simulink model "IFSSIM_Chassis"  (R2025b)
settings: Solver=FixedStepDiscrete  StartTime=0  StopTime=inf  FixedStep=1/960  RelTol=1e-3
undefined symbols (not defined in the file or in its folder): IFSSIM_CoGH, IFSSIM_Ixx, IFSSIM_Iyy, IFSSIM_Izz, IFSSIM_Mass, IFSSIM_Ts
settings Model: Creator=raulmoran  LastModifiedBy=raulmoran

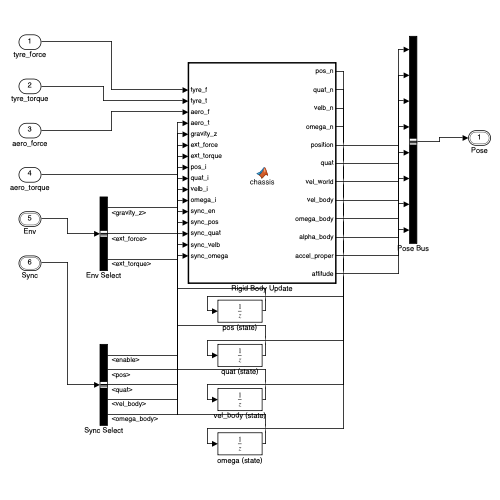
[thumbnail: Simulink's stored preview of the top-level diagram]
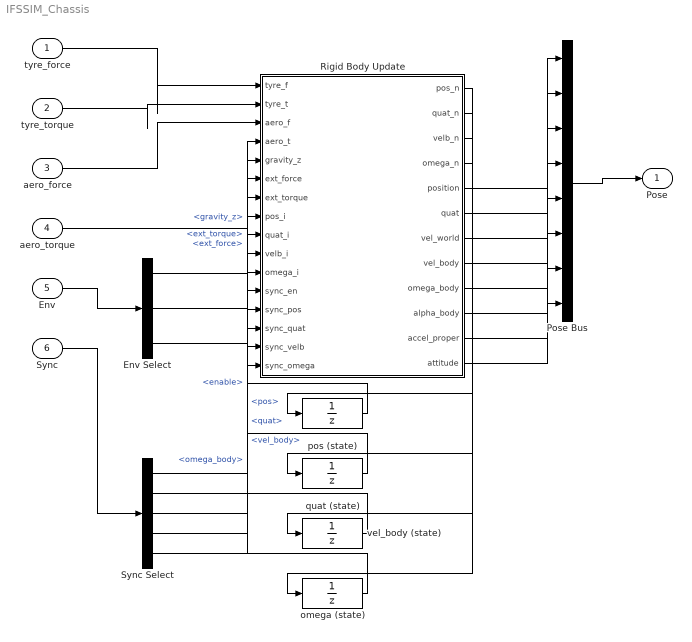
== system IFSSIM_Chassis ==
  tyre_force : Inport  PortDimensions=3
  tyre_torque : Inport  Port=2  PortDimensions=3
  aero_force : Inport  Port=3  PortDimensions=3
  aero_torque : Inport  Port=4  PortDimensions=3
  Env : Inport  Port=5  OutDataTypeStr=Bus: IFSSIM_EnvBus  BusOutputAsStruct=on
  Sync : Inport  Port=6  OutDataTypeStr=Bus: IFSSIM_SyncBus  BusOutputAsStruct=on
  Env Select : BusSelector  OutputSignals=gravity_z,ext_force,ext_torque
  Pose Bus : BusCreator  Inputs=8  OutDataTypeStr=Bus: IFSSIM_PoseBus  NonVirtualBus=on
  Rigid Body Update : MATLAB Function  TreatAsAtomicUnit=on
  Sync Select : BusSelector  OutputSignals=enable,pos,quat,vel_body,omega_body
  omega (state) : UnitDelay  InitialCondition=[0;0;0]  SampleTime=-1  HasFrameUpgradeWarning=on
  pos (state) : UnitDelay  InitialCondition=[0;0;IFSSIM_CoGH]  SampleTime=-1  HasFrameUpgradeWarning=on
  quat (state) : UnitDelay  InitialCondition=[1;0;0;0]  SampleTime=-1  HasFrameUpgradeWarning=on
  vel_body (state) : UnitDelay  InitialCondition=[0;0;0]  SampleTime=-1  HasFrameUpgradeWarning=on
  Pose : Outport  OutDataTypeStr=Bus: IFSSIM_PoseBus
  wires:
  Env/1 -> Env Select/1
  Sync/1 -> Sync Select/1
  Pose Bus/1 -> Pose/1
  tyre_force/1 -> Rigid Body Update/1(tyre_f)
  tyre_torque/1 -> Rigid Body Update/2(tyre_t)
  aero_force/1 -> Rigid Body Update/3(aero_f)
  aero_torque/1 -> Rigid Body Update/4(aero_t)
  Env Select/1 -> Rigid Body Update/5(gravity_z)  "<gravity_z>"
  Env Select/2 -> Rigid Body Update/6(ext_force)  "<ext_force>"
  Env Select/3 -> Rigid Body Update/7(ext_torque)  "<ext_torque>"
  pos (state)/1 -> Rigid Body Update/8(pos_i)
  quat (state)/1 -> Rigid Body Update/9(quat_i)
  vel_body (state)/1 -> Rigid Body Update/10(velb_i)
  omega (state)/1 -> Rigid Body Update/11(omega_i)
  Sync Select/1 -> Rigid Body Update/12(sync_en)  "<enable>"
  Sync Select/2 -> Rigid Body Update/13(sync_pos)  "<pos>"
  Sync Select/3 -> Rigid Body Update/14(sync_quat)  "<quat>"
  Sync Select/4 -> Rigid Body Update/15(sync_velb)  "<vel_body>"
  Sync Select/5 -> Rigid Body Update/16(sync_omega)  "<omega_body>"
  Rigid Body Update/1(pos_n) -> pos (state)/1
  Rigid Body Update/2(quat_n) -> quat (state)/1
  Rigid Body Update/3(velb_n) -> vel_body (state)/1
  Rigid Body Update/4(omega_n) -> omega (state)/1
  Rigid Body Update/5(position) -> Pose Bus/1
  Rigid Body Update/6(quat) -> Pose Bus/2
  Rigid Body Update/7(vel_world) -> Pose Bus/3
  Rigid Body Update/8(vel_body) -> Pose Bus/4
  Rigid Body Update/9(omega_body) -> Pose Bus/5
  Rigid Body Update/10(alpha_body) -> Pose Bus/6
  Rigid Body Update/11(accel_proper) -> Pose Bus/7
  Rigid Body Update/12(attitude) -> Pose Bus/8

== matlab function IFSSIM_Chassis/Rigid Body Update ==
  data: tyre_f input size=3; pos_n output size=3; tyre_t input size=3; aero_f input size=3; aero_t input size=3; gravity_z input size=1; ext_force input size=3; ext_torque input size=3; pos_i input size=3; quat_i input size=4; velb_i input size=3; omega_i input size=3; sync_en input size=1; sync_pos input size=3; sync_quat input size=4; sync_velb input size=3; sync_omega input size=3; quat_n output size=4; velb_n output size=3; omega_n output size=3; position output size=3; quat output size=4; vel_world output size=3; vel_body output size=3; omega_body output size=3; alpha_body output size=3; accel_proper output size=3; attitude output size=3; IFSSIM_Ts parameter size=1; IFSSIM_Mass parameter size=1; IFSSIM_Ixx parameter size=1; IFSSIM_Iyy parameter size=1; IFSSIM_Izz parameter size=1; IFSSIM_CoGH parameter size=1
function [pos_n, quat_n, velb_n, omega_n, position, quat, vel_world, vel_body, omega_body, alpha_body, accel_proper, attitude] = ...
         chassis(tyre_f, tyre_t, aero_f, aero_t, gravity_z, ext_force, ext_torque, pos_i, quat_i, velb_i, omega_i, ...
                 sync_en, sync_pos, sync_quat, sync_velb, sync_omega, IFSSIM_Ts, IFSSIM_Mass, IFSSIM_Ixx, IFSSIM_Iyy, IFSSIM_Izz, IFSSIM_CoGH)
%#codegen
% 6-DOF rigid body, Newton-Euler in the body frame, forward Euler at Ts.
%
% Frames: body is ISO 8855 / REP-103 — x forward, y LEFT, z up. World is ENU.
% Wheel order elsewhere is FL, FR, RL, RR.
%
% tyre_f / aero_f arrive in the BODY frame (they are generated by body-attached
% things). ext_force is WORLD — it comes from the platform's collision solver,
% which has no opinion about the car's orientation.
%
% The Env bus is split by a Bus Selector OUTSIDE this block rather than passed
% in whole. Two reasons: a MATLAB Function block has to infer a struct type
% through the port, which is fragile; and the selector makes the diagram show
% exactly which Env fields the chassis consumes.

% Flat workspace scalars, not IFSSIM_P.Assumed.Izz: a MATLAB Function block
% resolves workspace variables as parameters and that lookup does not reach
% into nested structs. See ifssim_load_workspace.m — still one source, still
% settings.json.
Ts = IFSSIM_Ts;
m  = IFSSIM_Mass;
I  = [IFSSIM_Ixx; IFSSIM_Iyy; IFSSIM_Izz];   % principal, diagonal

% --- state injection -------------------------------------------------
% Applied to the INCOMING state, before any dynamics. Overriding the outgoing
% state instead would look equivalent and is not: this step would still
% compute its forces and its reported acceleration from the OLD pose, so the
% caller would read a response to a state the plant is no longer in. For a
% one-step comparison against a reference that is precisely the wrong answer,
% and it is wrong by one step, which is the hardest kind of wrong to see.
%
% Normal running leaves enable at zero and nothing here executes.
if sync_en > 0.5
    pos_i   = sync_pos;
    quat_i  = sync_quat / max(norm(sync_quat), eps);
    velb_i  = sync_velb;
    omega_i = sync_omega;
end

% --- orientation ---------------------------------------------------
q = quat_i / max(norm(quat_i), eps);        % renormalise every step: forward Euler
                                        % on a quaternion drifts off the unit
                                        % sphere, and the drift is silent.
R = quat2rotm_local(q);                 % body -> world

% --- forces ----------------------------------------------------------
% Everything to the body frame first, then one sum. Mixing frames in a
% force accumulator is the classic way to get a plausible-but-wrong plant.
F_body = tyre_f + aero_f + R' * ext_force;
M_body = tyre_t + aero_t + R' * ext_torque;

% PROPER acceleration excludes gravity — it is what an accelerometer reads.
% Publishing this directly is the point: the simulator currently finite-
% differences a world velocity and bolts +g on, which is where the missing
% Coriolis terms in the EKF came from.
accel_proper = F_body / m;

% Gravity acts on the body but is NOT felt by an accelerometer, so it enters
% the equation of motion after accel_o has been taken.
g_body = R' * [0; 0; gravity_z];

% --- rigid body ------------------------------------------------------
% v_dot = F/m + g - omega x v      (Coriolis term: body-frame rates are not
%                                   inertial, and dropping this is exactly the
%                                   bug that made vy drift during cornering)
vdot  = accel_proper + g_body - cross(omega_i, velb_i);

% I*omega_dot = M - omega x (I*omega)   (gyroscopic coupling)
Iw    = I .* omega_i;
alpha_body = (M_body - cross(omega_i, Iw)) ./ I;

% --- integrate -------------------------------------------------------
velb_n  = velb_i + Ts * vdot;
omega_n = omega_i + Ts * alpha_body;

% Position integrates the WORLD velocity.
vel_world = R * velb_i;
pos_n   = pos_i + Ts * vel_world;

% q_dot = 0.5 * q (x) [0; omega]
qd      = 0.5 * quatmul_local(q, [0; omega_i]);
quat_n  = q + Ts * qd;
quat_n  = quat_n / max(norm(quat_n), eps);

% --- reported state ---------------------------------------------------
position = pos_i;
quat    = q;
vel_body = velb_i;
omega_body = omega_i;

% attitude = [roll; pitch; heave]. Heave is height above the declared static
% CoG height, so 0 means sitting at ride height rather than at the world origin.
roll_  = atan2(2*(q(1)*q(2) + q(3)*q(4)), 1 - 2*(q(2)^2 + q(3)^2));
sinp   = 2*(q(1)*q(3) - q(4)*q(2));
pitch_ = asin(max(-1, min(1, sinp)));
attitude = [roll_; pitch_; pos_i(3) - IFSSIM_CoGH];
end

function R = quat2rotm_local(q)
%#codegen
w = q(1); x = q(2); y = q(3); z = q(4);
R = [1-2*(y*y+z*z),   2*(x*y-z*w),   2*(x*z+y*w); ...
       2*(x*y+z*w), 1-2*(x*x+z*z),   2*(y*z-x*w); ...
       2*(x*z-y*w),   2*(y*z+x*w), 1-2*(x*x+y*y)];
end

function r = quatmul_local(a, b)
%#codegen
r = [a(1)*b(1) - a(2)*b(2) - a(3)*b(3) - a(4)*b(4); ...
     a(1)*b(2) + a(2)*b(1) + a(3)*b(4) - a(4)*b(3); ...
     a(1)*b(3) - a(2)*b(4) + a(3)*b(1) + a(4)*b(2); ...
     a(1)*b(4) + a(2)*b(3) - a(3)*b(2) + a(4)*b(1)];
end
